simulink model "Model_Following_Destrete"  (Simulink 8.4)
settings: Solver=ode45  StartTime=0.0  StopTime=10.0  RelTol=1e-3
values from neighbouring files (symbols this model uses):
  A = [0 0 0 0 0 226436.678287 -162511.258811 0 0 0 0 0 ... (100 elements, 10x10)]    [AMB_discrete_parameter.mat]    (also in OKID_AMBsystem_discrete_XY.m = [zeros(4) eye(4); Ae Ag]; OKID_AMBsystem_discrete_Z.m = [zeros(1) eye(1); Ae Ag]; era_WT.m = Sigma^(-0.5)*U'*H1*V*Sigma^(-0.5); sys_XY.mat = [0 0 0 0 226436.678287 -162511.258811 0 0 0 0 0 0 ... (64 el)
  B = [0 0 0 0 0 82.3406102861 -59.095003204 0 0 0 0 0 ... (50 elements, 10x5)]    [AMB_discrete_parameter.mat]    (also in OKID_AMBsystem_discrete_XY.m = [zeros(4); Bi]; OKID_AMBsystem_discrete_Z.m = [zeros(1); Bi]; era_WT.m = Btemp(:, 1:r); sys_XY.mat = [0 0 0 0 82.3406102861 -59.095003204 0 0 0 0 0 0 ... (32 ele)
  C = [1 -1.11022302463e-16 0 0 0 -5.55111512313e-17 1 0 0 0 0 0 ... (50 elements, 5x10)]    [AMB_discrete_parameter.mat]    (also in OKID_AMBsystem_discrete_XY.m = [Ci*inv(T') zeros(4)]; OKID_AMBsystem_discrete_Z.m = [Ci*inv(T') zeros(1)]; era_WT.m = Ctemp(1:m, :); sys_XY.mat = [1 -1.11022302463e-16 0 0 -5.55111512313e-17 1 0 0 0 0 1 -1.)
  Cd = 0    [AMB_5DOF_Destrete.m]    (also in AMB_discrete_parameter.mat = [-1.86122185924e-05 -1.53395990555e-05 0.340435639158 0.2963)
  Cu_star = inv(Rd_wave)*(H'*inv((G-H*Kd)'-eye(nr))*Kd'+eye(mr))*Rd    [AMB_5DOF_Destrete.m]    (also in AMB_discrete_parameter.mat = [-0.0660333645837 -0.00684036739434 -0.000550867351687 0.000)
  D = zeros(size(C,1),size(B,2))    [AMB_5DOF_Destrete.m]    (also in AMB_discrete_parameter.mat = [0 0 0 0 0 0 0 0 0 0 0 0 ... (25 elements, 5x5)]; OKID_AMBsystem_discrete_XY.m = zeros(pr,mr); OKID_AMBsystem_discrete_Z.m = zeros(pr,mr))
  Ed = inv(Rd_wave)*(D'+H'*inv(eye(nr)-(G-H*Kd)')*(C_ok-D*Kd)')*Qd    [AMB_5DOF_Destrete.m]    (also in AMB_discrete_parameter.mat = [24012.1325759 2487.40632521 200.315400614 -209.616880608 0 )
  Kd = [26943.7243285 2506.21733555 201.830285154 -211.202108856 0 2507.80191387 26050.0887338 349.151630032 -386.670927976 0 -417.194546257 -457.001698507 ... (50 elements, 5x10)]    [AMB_discrete_parameter.mat]
  Ts = 0.00025    [AMB_discrete_parameter.mat]    (also in OKID_AMBsystem_discrete_XY.m = 1e-06; OKID_AMBsystem_discrete_Z.m = 0.01; sys_XY.mat = 1e-06)
  ud_star = [0 0 0 0]'    [AMB_5DOF_Destrete.m]    (also in AMB_discrete_parameter.mat = [0 0 0 0 0])
  x = [0 0 0 0 0 0 0 0 0 0]    [AMB_discrete_parameter.mat]    (also in OKID_AMBsystem_discrete_XY.m = zeros(nr,1); OKID_AMBsystem_discrete_Z.m = zeros(nr,1))
settings Model: Creator=koni  LastModifiedBy=123  CovSFcnEnable=on
settings DebuggingCC: FrameProcessingCompatibilityMsg=error

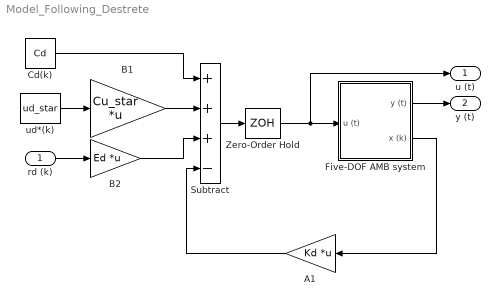
== system Model_Following_Destrete ==
  rd (k) : Inport  PortDimensions=pr
  " Five-DOF AMB system" : Subsystem
  A1 : Gain  Gain=Kd  Multiplication=Matrix(K*u)
  B1 : Gain  Gain=Cu_star  Multiplication=Matrix(K*u)
  B2 : Gain  Gain=Ed  Multiplication=Matrix(K*u)
  Cd(k) : Constant  Value=Cd
  Subtract : Sum  Inputs=+++-
  Zero-Order Hold : ZeroOrderHold  SampleTime=Ts
  ud*(k) : Constant  Value=ud_star
  u (t) : Outport  PortDimensions=mr
  y (t) : Outport  Port=2  PortDimensions=pr
  wires:
  " Five-DOF AMB system"/1(y (t)) -> y (t)/1
  Subtract/1 -> Zero-Order Hold/1
  B2/1 -> Subtract/3
  rd (k)/1 -> B2/1
  " Five-DOF AMB system"/2(x (k)) -> A1/1
  A1/1 -> Subtract/4
  ud*(k)/1 -> B1/1
  B1/1 -> Subtract/2
  Cd(k)/1 -> Subtract/1
  Zero-Order Hold/1 -> " Five-DOF AMB system"/1(u (t)), u (t)/1

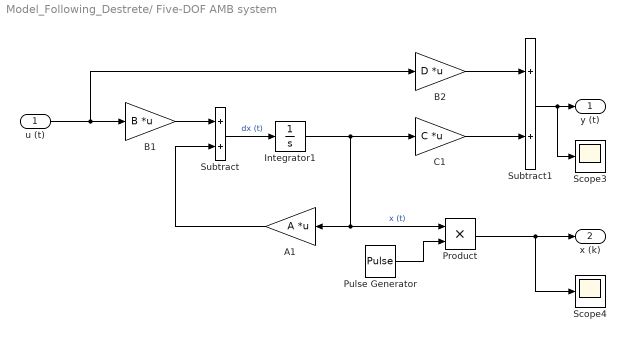
== system Model_Following_Destrete/ Five-DOF AMB system ==
  u (t) : Inport  PortDimensions=mr
  A1 : Gain  Gain=A  Multiplication=Matrix(K*u)
  B1 : Gain  Gain=B  Multiplication=Matrix(K*u)
  B2 : Gain  Gain=D  Multiplication=Matrix(K*u)
  C1 : Gain  Gain=C  Multiplication=Matrix(K*u)
  Integrator1 : Integrator  InitialCondition=x(:,1)
  Product : Product
  Pulse Generator : DiscretePulseGenerator  PulseType=Time based  Period=Ts
  Scope3 : Scope
      settings: TimeRange=0.05  SaveName=ScopeData2
  Scope4 : Scope
      settings: TimeRange=0.04999  YMin=-0.001  YMax=0.006  SaveName=ScopeData3
  Subtract : Sum
  Subtract1 : Sum
  y (t) : Outport  PortDimensions=pr
  x (k) : Outport  Port=2  PortDimensions=nr
  wires:
  Subtract/1 -> Integrator1/1  "dx (t)"
  Integrator1/1 -> C1/1, A1/1, Product/1  "x (t)"
  u (t)/1 -> B1/1, B2/1
  B1/1 -> Subtract/1
  A1/1 -> Subtract/2
  Subtract1/1 -> Scope3/1, y (t)/1
  C1/1 -> Subtract1/2
  B2/1 -> Subtract1/1
  Product/1 -> Scope4/1, x (k)/1
  Pulse Generator/1 -> Product/2
